simulink model "mrac_lyap"  (R2020b)
settings: Solver=VariableStepAuto  StartTime=0.0  StopTime=10.0  RelTol=1e-3
values from neighbouring files (symbols this model uses):
  am = -4    [init_mrac.m]    (also in init_mraclb.m = [0 1; -wn^2 -2*zet*wn])
  ao = [0 1; thet1o thet2o]    [init_mraclb.m]
  bbo = [0; 1]    [init_mraclb.m]
  bm = 4    [init_mrac.m]    (also in init_mraclb.m = [0; wn^2])
  cm = [1 0; 0 1]    [init_mraclb.m]
  dm = [0; 0]    [init_mraclb.m]
  gphi_i = 2000*eye(3)    [init_mraclb.m]
  gr_i = 2000    [init_mraclb.m]
  gx_i = 2000*eye(2)    [init_mraclb.m]
  Ko = [k1o; k2o]    [init_mraclb.m]
  lo = wn^2/thet6o    (= 5.33333333333)    [init_mraclb.m]
  P = eye(2)*1000    [init_miac.m]    (also in init_mraclb.m = lyap(am,Q); miac_rls2.m = P - (P*(phi*phi')*P)/(1+phi'*P*phi))
  thet3o = -0.062    [init_mraclb.m]
  thet4o = 0.009    [init_mraclb.m]
  thet5o = 0.021    [init_mraclb.m]
  thet6o = 0.75    [init_mraclb.m]
  Thetao = [thet3o/thet6o; thet4o/thet6o; thet5o/thet6o]    [init_mraclb.m]
settings Model: Creator=Melkamu A  LastModifiedBy=Melkamu A

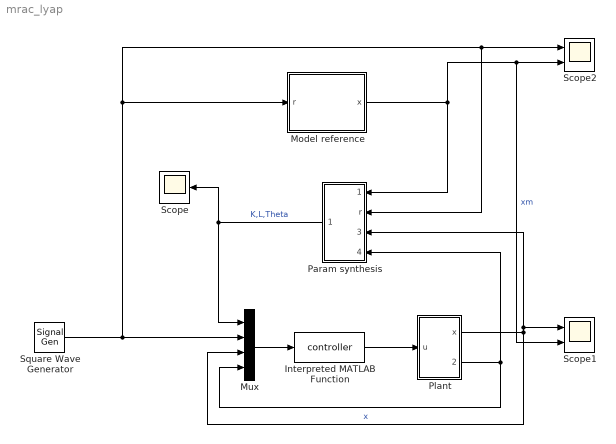
== system mrac_lyap ==
  Interpreted MATLAB Function : MATLABFcn  MATLABFcn=controller  OutputDimensions=1
  Model reference : Subsystem
  Mux : Mux  Inputs=[6 1 2 3]
  Param synthesis : Subsystem
  Plant : Subsystem
  Scope : Scope
  Scope1 : Scope  NumInputPorts=2
  Scope2 : Scope  NumInputPorts=2
  Square Wave Generator : SignalGenerator  WaveForm=square  Amplitude=0.3  Frequency=0.25
  wires:
  Interpreted MATLAB Function/1 -> Plant/1(u)
  Mux/1 -> Interpreted MATLAB Function/1
  Model reference/1(x) -> Param synthesis/1(xm), Scope1/2, Scope2/2  "xm"
  Plant/1(x) -> Scope1/1, Param synthesis/3(In3), Mux/3  "x"
  Plant/2(phi_x) -> Mux/4, Param synthesis/4(In4)
  Param synthesis/1(Out1) -> Scope/1, Mux/1  "K,L,Theta"
  Square Wave Generator/1 -> Mux/2, Model reference/1(r), Param synthesis/2(r), Scope2/1

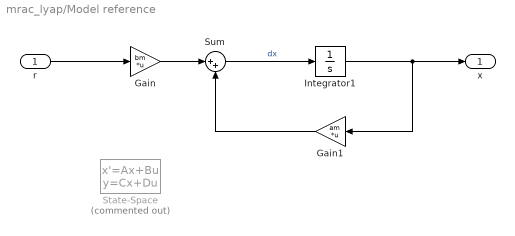
== system mrac_lyap/Model reference ==
  r : Inport
  Gain : Gain  Gain=bm  Multiplication=Matrix(K*u)
  Gain1 : Gain  Gain=am  Multiplication=Matrix(K*u)
  Integrator1 : Integrator
  State-Space : StateSpace  Commented=on  A=am  B=bm  C=cm  D=dm  InitialCondition=0
  Sum : Sum  Inputs=|++
  x : Outport
  wires:
  Integrator1/1 -> Gain1/1, x/1
  Gain1/1 -> Sum/2
  Sum/1 -> Integrator1/1  "dx"
  Gain/1 -> Sum/1
  r/1 -> Gain/1

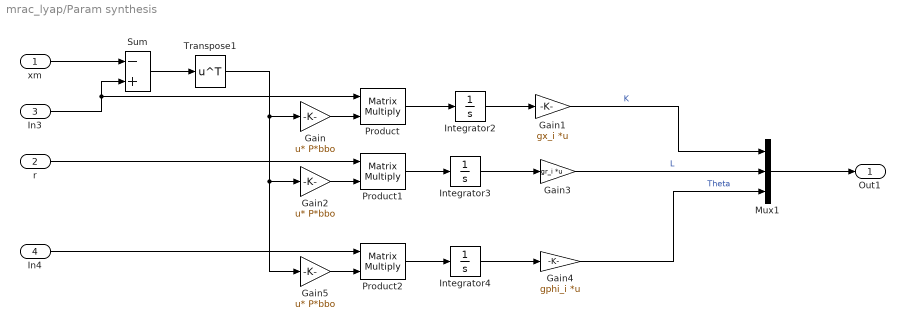
== system mrac_lyap/Param synthesis ==
  xm : Inport
  r : Inport  Port=2
  In3 : Inport  Port=3
  In4 : Inport  Port=4
  Gain : Gain  Gain=P*bbo  Multiplication=Matrix(u*K)
  Gain1 : Gain  Gain=gx_i  Multiplication=Matrix(K*u)
  Gain2 : Gain  Gain=P*bbo  Multiplication=Matrix(u*K)
  Gain3 : Gain  Gain=gr_i  Multiplication=Matrix(K*u)
  Gain4 : Gain  Gain=gphi_i  Multiplication=Matrix(K*u)
  Gain5 : Gain  Gain=P*bbo  Multiplication=Matrix(u*K)
  Integrator2 : Integrator  InitialCondition=Ko
  Integrator3 : Integrator  InitialCondition=lo
  Integrator4 : Integrator  InitialCondition=Thetao
  Mux1 : Mux  Inputs=[2 1 3]
  Product : Product  Multiplication=Matrix(*)
  Product1 : Product  Multiplication=Matrix(*)
  Product2 : Product  Multiplication=Matrix(*)
  Sum : Sum  Inputs=-+
  Transpose1 : Math  Operator=transpose  SaturateOnIntegerOverflow=on
  Out1 : Outport
  wires:
  Gain3/1 -> Mux1/2  "L"
  Sum/1 -> Transpose1/1
  Integrator4/1 -> Gain4/1
  Transpose1/1 -> Gain5/1, Gain2/1, Gain/1
  Integrator3/1 -> Gain3/1
  Gain1/1 -> Mux1/1  "K"
  Integrator2/1 -> Gain1/1
  In3/1 -> Sum/2, Product/1
  Product/1 -> Integrator2/1
  xm/1 -> Sum/1
  Gain4/1 -> Mux1/3  "Theta"
  Mux1/1 -> Out1/1
  Product1/1 -> Integrator3/1
  r/1 -> Product1/1
  Product2/1 -> Integrator4/1
  Gain5/1 -> Product2/2
  In4/1 -> Product2/1
  Gain2/1 -> Product1/2
  Gain/1 -> Product/2

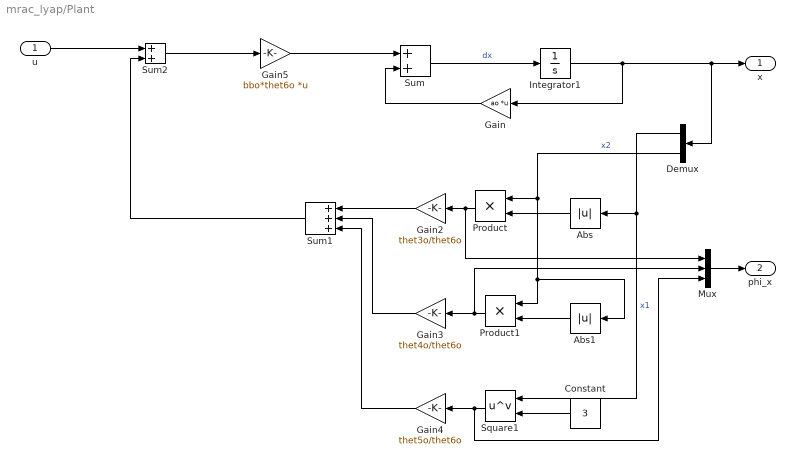
== system mrac_lyap/Plant ==
  u : Inport
  Abs : Abs
  Abs1 : Abs
  Constant : Constant  Value=3
  Demux : Demux  Outputs=2
  Gain : Gain  Gain=ao  Multiplication=Matrix(K*u)
  Gain2 : Gain  Gain=thet3o/thet6o
  Gain3 : Gain  Gain=thet4o/thet6o
  Gain4 : Gain  Gain=thet5o/thet6o
  Gain5 : Gain  Gain=bbo*thet6o  Multiplication=Matrix(K*u)
  Integrator1 : Integrator
  Mux : Mux  Inputs=3
  Product : Product
  Product1 : Product
  Square1 : Math  Operator=pow  SaturateOnIntegerOverflow=on
  Sum : Sum
  Sum1 : Sum  Inputs=+++
  Sum2 : Sum
  x : Outport
  phi_x : Outport  Port=2
  wires:
  Sum/1 -> Integrator1/1  "dx"
  Gain3/1 -> Sum1/2
  Product/1 -> Mux/1, Gain2/1
  Sum1/1 -> Sum2/2
  Gain5/1 -> Sum/1
  Constant/1 -> Square1/2
  Gain4/1 -> Sum1/3
  Integrator1/1 -> Gain/1, Demux/1, x/1
  Gain2/1 -> Sum1/1
  Gain/1 -> Sum/2
  Sum2/1 -> Gain5/1
  u/1 -> Sum2/1
  Product1/1 -> Mux/2, Gain3/1
  Abs1/1 -> Product1/2
  Abs/1 -> Product/2
  Square1/1 -> Mux/3, Gain4/1
  Mux/1 -> phi_x/1
  Demux/2 -> Product1/1, Abs1/1, Product/1  "x2"
  Demux/1 -> Square1/1, Abs/1  "x1"
